simulink model "motor_stateback"  (R2018b)
settings: Solver=FixedStepAuto  StartTime=0.0  StopTime=10.0  FixedStep=0.001  RelTol=1e-3
values from neighbouring files (symbols this model uses):
  k1 = (wn^2 - 98)/(-100)    (= -0.02)    [Para_stateback.m]
  k2 = (2 - 2*xigemamax*wn)/(100)    [Para_stateback.m]
settings Model: Creator=chengqian  LastModifiedBy=chengqian
settings OptimizationCC: DefaultParameterBehavior=Inlined  BufferReuse=off
settings DebuggingCC: InitInArrayFormatMsg=none

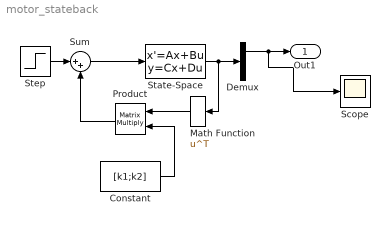
== system motor_stateback ==
  Constant : Constant  Value=[k1;k2]
  Demux : Demux  Outputs=2
  Math Function : Math  Operator=transpose  SaturateOnIntegerOverflow=on
  Product : Product  Multiplication=Matrix(*)
  Scope : Scope
  State-Space : StateSpace  A=[0,1;-98,-2]  B=[0;100]  C=eye(2)  D=[0;0]  InitialCondition=[0;0]
  Step : Step  Time=0  SampleTime=0
  Sum : Sum  Inputs=|++
  Out1 : Outport
  wires:
  Sum/1 -> State-Space/1
  Product/1 -> Sum/2
  Constant/1 -> Product/2
  State-Space/1 -> Math Function/1, Demux/1
  Math Function/1 -> Product/1
  Demux/1 -> Scope/1, Out1/1
  Step/1 -> Sum/1
